simulink model "swingupcontroller"  (R2019b)
settings: Solver=VariableStepAuto  StartTime=0.0  StopTime=10.0  RelTol=1e-3
values from neighbouring files (symbols this model uses):
  epsilon = 12.0 * pi / 180    (= 0.209439510239)    [ripbalanced.m]    (also in setup_rotpen.m)
  eta_g = 0.90    (= 0.9)    [config_servo.m]    (also in dripbalanced.m; ripbalanced.m; test_drip.m)
  eta_m = 0.69    [config_servo.m]    (also in dripbalanced.m; ripbalanced.m; test_drip.m)
  g = 9.81    [RIP_ABCD_SS.m]    (also in RIP_ABCD_SS_1.m; RIP_ABCD_SS_2.m; RIP_ABCD_SS_3.m; RIP_ABCD_SS_POLE_PLACE.m)
  Jp = 0.001198    [RIP_ABCD_SS.m]    (also in RIP_ABCD_SS_2.m = 0.0023; RIP_ABCD_SS_3.m; RIP_ABCD_SS_POLE_PLACE.m; Untitled3.m = 0.0012)
  K = [0 0 0 0]    [Pole_placement.m]    (also in RIP_ABCD_SS.m = lqr(A,B,Q,R); RIP_ABCD_SS_POLE_PLACE.m = lqr(A,B,Q,R); ripbalanced.m = acker(A,B,DP); setup_rotpen.m = d_balance(A, B, zeta, wn, p3, p4))
  K_AMP = 1    [dripbalanced.m]    (also in ripbalanced.m; setup_rotpen.m; test_drip.m)
  Kg = 70    [RIP_ABCD_SS.m]    (also in RIP_ABCD_SS_1.m = 14; RIP_ABCD_SS_2.m; RIP_ABCD_SS_3.m; RIP_ABCD_SS_POLE_PLACE.m)
  km = 0.007677    [RIP_ABCD_SS.m]    (also in RIP_ABCD_SS_1.m = 0.00767; RIP_ABCD_SS_2.m = 0.00767; RIP_ABCD_SS_3.m; RIP_ABCD_SS_POLE_PLACE.m)
  kt = 0.007682    [RIP_ABCD_SS.m]    (also in RIP_ABCD_SS_1.m = 0.00767; RIP_ABCD_SS_2.m = 0.00767; RIP_ABCD_SS_3.m; RIP_ABCD_SS_POLE_PLACE.m)
  Lp = 0.33655    [RIP_ABCD_SS.m]    (also in RIP_ABCD_SS_1.m = 0.337; RIP_ABCD_SS_2.m = 0.6413; RIP_ABCD_SS_3.m; RIP_ABCD_SS_POLE_PLACE.m)
  Lr = 0.2159    [RIP_ABCD_SS.m]    (also in RIP_ABCD_SS_1.m = 0.216; RIP_ABCD_SS_2.m; RIP_ABCD_SS_3.m; RIP_ABCD_SS_POLE_PLACE.m)
  Mp = 0.127    [RIP_ABCD_SS.m]    (also in RIP_ABCD_SS_1.m; RIP_ABCD_SS_2.m = 0.23; RIP_ABCD_SS_3.m; RIP_ABCD_SS_POLE_PLACE.m)
  Mr = 0.257    [RIP_ABCD_SS.m]    (also in RIP_ABCD_SS_3.m; RIP_ABCD_SS_POLE_PLACE.m; dripbalanced.m; ripbalanced.m)
  Rm = 2.6    [RIP_ABCD_SS.m]    (also in RIP_ABCD_SS_1.m; RIP_ABCD_SS_2.m; RIP_ABCD_SS_3.m; RIP_ABCD_SS_POLE_PLACE.m)
libraries: simulink_extras x3, simulink x3
settings Model: Creator=Ridma  LastModifiedBy=Ridma

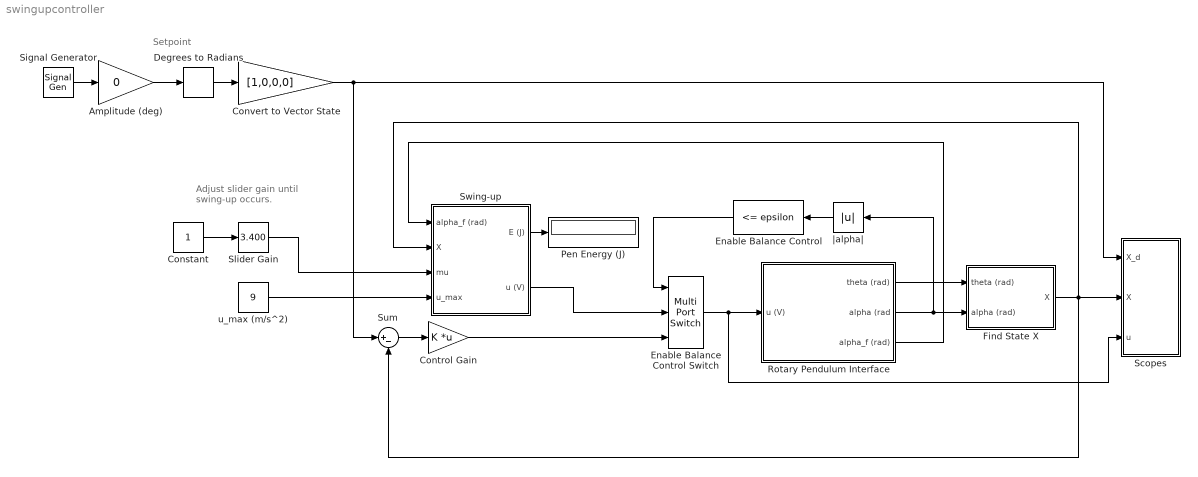
== system swingupcontroller ==
  note: Adjust slider gain
      | until swing-up occurs.
  note: Setpoint
  Amplitude (deg) : Gain  Gain=0  SaturateOnIntegerOverflow=on  OutDataTypeStr=Inherit: Same as input  ParamDataTypeStr=Inherit: Same as input
  Constant : Constant
  Control Gain : Gain  Gain=K  Multiplication=Matrix(K*u)
  Convert to Vector State : Gain  Gain=[1,0,0,0]
  Degrees to Radians : simulink_extras/Transformations/Degrees to Radians
  Enable Balance Control : simulink/Logic and Bit Operations/Compare To Constant  relop=<=  const=epsilon  OutDataTypeStr=uint8  ZeroCross=off
  Enable Balance Control Switch : MultiPortSwitch  DataPortOrder=Zero-based contiguous  Inputs=2  zeroidx=on
  Find State X : Subsystem
  Pen Energy (J) : Display
      settings: Decimation=100
  Rotary Pendulum Interface : Subsystem
  Scopes : Subsystem
  Signal Generator : SignalGenerator  WaveForm=square  Frequency=0.1
  Slider Gain : simulink/Math Operations/Slider Gain  gain=3.400  low=0  high=10
  Sum : Sum  Inputs=|+-
  Swing-up : Subsystem
  u_max (m/s^2) : Constant  Value=9
  |alpha| : Abs
  wires:
  Enable Balance Control Switch/1 -> Rotary Pendulum Interface/1(u (V)), Scopes/3(u)
  Control Gain/1 -> Enable Balance Control Switch/3
  Enable Balance Control/1 -> Enable Balance Control Switch/1
  Rotary Pendulum Interface/2(alpha (rad) -> Find State X/2(alpha (rad)), |alpha|/1
  Sum/1 -> Control Gain/1
  Constant/1 -> Slider Gain/1
  |alpha|/1 -> Enable Balance Control/1
  Rotary Pendulum Interface/3(alpha_f (rad)) -> Swing-up/1(alpha_f (rad))
  Swing-up/2(u (V)) -> Enable Balance Control Switch/2
  Slider Gain/1 -> Swing-up/3(mu)
  Swing-up/1(E (J)) -> Pen Energy (J)/1
  Signal Generator/1 -> Amplitude (deg)/1
  u_max (m/s^2)/1 -> Swing-up/4(u_max)
  Rotary Pendulum Interface/1(theta (rad)) -> Find State X/1(theta (rad))
  Find State X/1(X) -> Scopes/2(X), Sum/2, Swing-up/2(X)
  Convert to Vector State/1 -> Scopes/1(X_d), Sum/1
  Degrees to Radians/1 -> Convert to Vector State/1
  Amplitude (deg)/1 -> Degrees to Radians/1

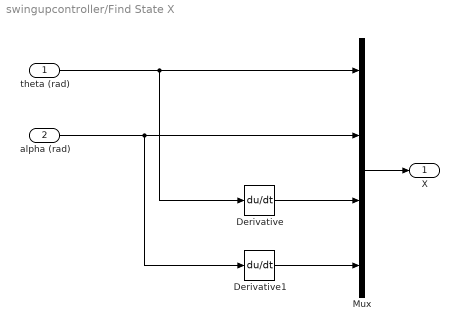
== system swingupcontroller/Find State X ==
  theta (rad) : Inport
  alpha (rad) : Inport  Port=2
  Derivative : Derivative
  Derivative1 : Derivative
  Mux : Mux
  X : Outport  VectorParamsAs1DForOutWhenUnconnected=off
  wires:
  alpha (rad)/1 -> Derivative1/1, Mux/2
  Mux/1 -> X/1
  theta (rad)/1 -> Derivative/1, Mux/1
  Derivative/1 -> Mux/3
  Derivative1/1 -> Mux/4

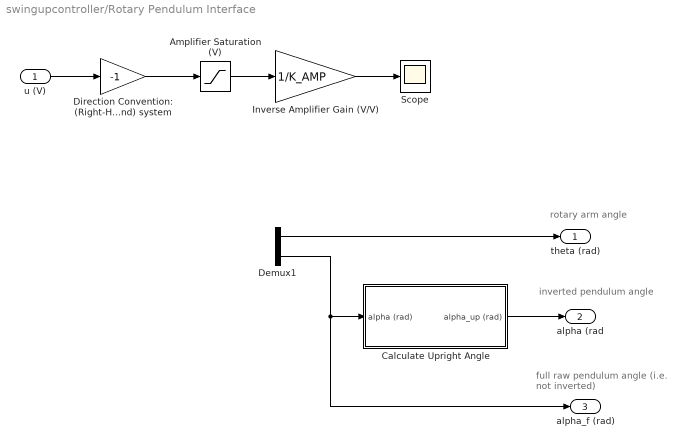
== system swingupcontroller/Rotary Pendulum Interface ==
  note: full raw pendulum angle
      |  (i.e. not inverted)
  note: rotary arm angle
  note: inverted pendulum angle
  u (V) : Inport
  Amplifier Saturation (V) : Saturate  UpperLimit=5  LowerLimit=-5
  Calculate Upright Angle : Subsystem
  Demux1 : Demux  Outputs=2
  Direction Convention: (Right-Hand) system : Gain  Gain=-1  SaturateOnIntegerOverflow=on  OutDataTypeStr=Inherit: Same as input  ParamDataTypeStr=Inherit: Same as input
  Inverse Amplifier Gain (V/V) : Gain  Gain=1/K_AMP
  Scope : Scope
  theta (rad) : Outport  VectorParamsAs1DForOutWhenUnconnected=off
  alpha (rad : Outport  Port=2  VectorParamsAs1DForOutWhenUnconnected=off
  alpha_f (rad) : Outport  Port=3  VectorParamsAs1DForOutWhenUnconnected=off
  wires:
  Calculate Upright Angle/1(alpha_up (rad)) -> alpha (rad/1
  Demux1/1 -> theta (rad)/1
  Direction Convention: (Right-Hand) system/1 -> Amplifier Saturation (V)/1
  u (V)/1 -> Direction Convention: (Right-Hand) system/1
  Inverse Amplifier Gain (V/V)/1 -> Scope/1
  Amplifier Saturation (V)/1 -> Inverse Amplifier Gain (V/V)/1
  Demux1/2 -> alpha_f (rad)/1, Calculate Upright Angle/1(alpha (rad))

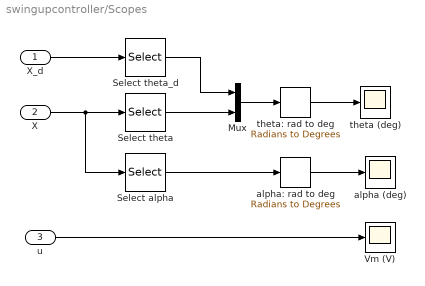
== system swingupcontroller/Scopes ==
  X_d : Inport
  X : Inport  Port=2
  u : Inport  Port=3
  Mux : Mux  Inputs=2
  Select alpha : Selector  InputPortWidth=4  IndexOptions=Index vector (dialog)  Indices=2  OutputSizes=[(-2)]
  Select theta : Selector  InputPortWidth=4  IndexOptions=Index vector (dialog)  Indices=1  OutputSizes=[(-2)]
  Select theta_d : Selector  InputPortWidth=4  IndexOptions=Index vector (dialog)  Indices=1  OutputSizes=[(-2)]
  Vm (V) : Scope
  alpha (deg) : Scope
  alpha: rad to deg : simulink_extras/Transformations/Radians to Degrees
  theta (deg) : Scope
  theta: rad to deg : simulink_extras/Transformations/Radians to Degrees
  wires:
  u/1 -> Vm (V)/1
  X_d/1 -> Select theta_d/1
  Mux/1 -> theta: rad to deg/1
  Select alpha/1 -> alpha: rad to deg/1
  alpha: rad to deg/1 -> alpha (deg)/1
  X/1 -> Select alpha/1, Select theta/1
  Select theta_d/1 -> Mux/1
  theta: rad to deg/1 -> theta (deg)/1
  Select theta/1 -> Mux/2

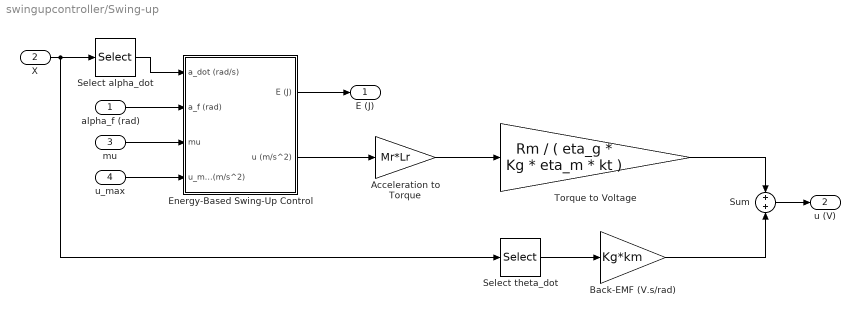
== system swingupcontroller/Swing-up ==
  alpha_f (rad) : Inport
  X : Inport  Port=2
  mu : Inport  Port=3
  u_max : Inport  Port=4
  Acceleration to Torque : Gain  Gain=Mr*Lr
  Back-EMF (V.s/rad) : Gain  Gain=Kg*km
  Energy-Based Swing-Up Control : Subsystem
  Select alpha_dot : Selector  InputPortWidth=4  IndexOptions=Index vector (dialog)  Indices=[4]  OutputSizes=1
  Select theta_dot : Selector  InputPortWidth=4  IndexOptions=Index vector (dialog)  Indices=[3]  OutputSizes=1
  Sum : Sum
  Torque to Voltage : Gain  Gain=Rm / ( eta_g * Kg * eta_m * kt )
  E (J) : Outport  VectorParamsAs1DForOutWhenUnconnected=off
  u (V) : Outport  Port=2  VectorParamsAs1DForOutWhenUnconnected=off
  wires:
  Energy-Based Swing-Up Control/2(u (m/s^2)) -> Acceleration to Torque/1
  Acceleration to Torque/1 -> Torque to Voltage/1
  Energy-Based Swing-Up Control/1(E (J)) -> E (J)/1
  alpha_f (rad)/1 -> Energy-Based Swing-Up Control/2(a_f (rad))
  mu/1 -> Energy-Based Swing-Up Control/3(mu)
  Select alpha_dot/1 -> Energy-Based Swing-Up Control/1(a_dot (rad/s))
  X/1 -> Select alpha_dot/1, Select theta_dot/1
  u_max/1 -> Energy-Based Swing-Up Control/4(u_max (m/s^2))
  Select theta_dot/1 -> Back-EMF (V.s/rad)/1
  Torque to Voltage/1 -> Sum/1
  Back-EMF (V.s/rad)/1 -> Sum/2
  Sum/1 -> u (V)/1

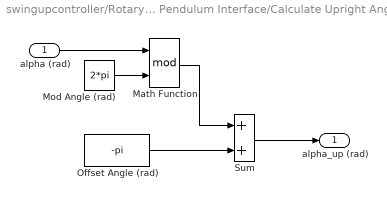
== system swingupcontroller/Rotary Pendulum Interface/Calculate Upright Angle ==
  alpha (rad) : Inport
  Math Function : Math  Operator=mod  SaturateOnIntegerOverflow=on
  Mod Angle (rad) : Constant  Value=2*pi
  Offset Angle (rad) : Constant  Value=-pi
  Sum : Sum  SaturateOnIntegerOverflow=on  InputSameDT=on  OutDataTypeStr=Inherit: Same as first input
  alpha_up (rad) : Outport  VectorParamsAs1DForOutWhenUnconnected=off
  wires:
  Math Function/1 -> Sum/1
  alpha (rad)/1 -> Math Function/1
  Offset Angle (rad)/1 -> Sum/2
  Mod Angle (rad)/1 -> Math Function/2
  Sum/1 -> alpha_up (rad)/1

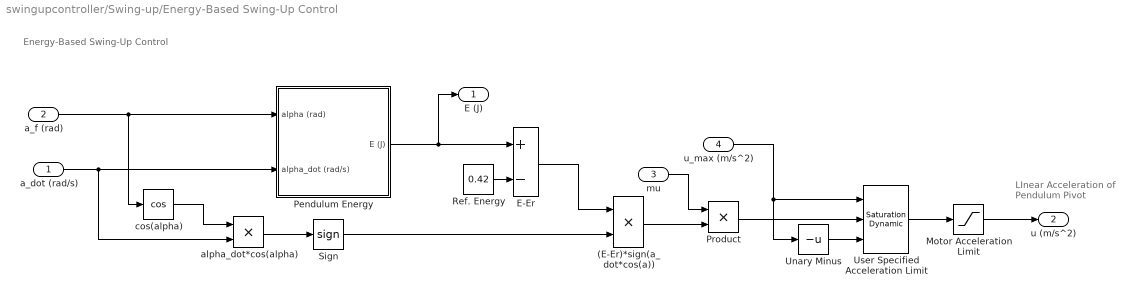
== system swingupcontroller/Swing-up/Energy-Based Swing-Up Control ==
  note: Energy-Based Swing-Up Control
  note: LInear Acceleration of
      | Pendulum Pivot
  a_dot (rad/s) : Inport
  a_f (rad) : Inport  Port=2
  mu : Inport  Port=3
  u_max (m/s^2) : Inport  Port=4
  (E-Er)*sign(a_dot*cos(a)) : Product  RndMeth=Zero
  E-Er : Sum  Inputs=+-
  Motor Acceleration Limit : Saturate  UpperLimit=9  LowerLimit=-9
  Pendulum Energy : Subsystem
  Product : Product  RndMeth=Zero
  Ref. Energy : Constant  Value=0.42
  Sign : Signum
  Unary Minus : UnaryMinus
  User Specified Acceleration Limit : simulink/Discontinuities/Saturation Dynamic  OutMin=[]  OutMax=[]  OutDataTypeStr=Inherit: Same as second input  OutDataType=fixdt(1, 16)  OutScaling=2^-10  DoSatur=off
  alpha_dot*cos(alpha) : Product  RndMeth=Zero
  cos(alpha) : Trigonometry  Operator=cos
  E (J) : Outport  VectorParamsAs1DForOutWhenUnconnected=off
  u (m/s^2) : Outport  Port=2  VectorParamsAs1DForOutWhenUnconnected=off
  wires:
  alpha_dot*cos(alpha)/1 -> Sign/1
  Sign/1 -> (E-Er)*sign(a_dot*cos(a))/2
  cos(alpha)/1 -> alpha_dot*cos(alpha)/1
  a_f (rad)/1 -> cos(alpha)/1, Pendulum Energy/1(alpha (rad))
  E-Er/1 -> (E-Er)*sign(a_dot*cos(a))/1
  Pendulum Energy/1(E (J)) -> E (J)/1, E-Er/1
  a_dot (rad/s)/1 -> alpha_dot*cos(alpha)/2, Pendulum Energy/2(alpha_dot (rad/s))
  (E-Er)*sign(a_dot*cos(a))/1 -> Product/2
  Ref. Energy/1 -> E-Er/2
  mu/1 -> Product/1
  Product/1 -> User Specified Acceleration Limit/2
  u_max (m/s^2)/1 -> User Specified Acceleration Limit/1, Unary Minus/1
  Unary Minus/1 -> User Specified Acceleration Limit/3
  User Specified Acceleration Limit/1 -> Motor Acceleration Limit/1
  Motor Acceleration Limit/1 -> u (m/s^2)/1

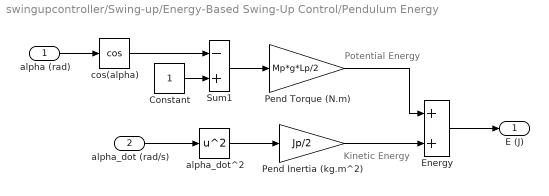
== system swingupcontroller/Swing-up/Energy-Based Swing-Up Control/Pendulum Energy ==
  note: Kinetic Energy
  note: Potential Energy
  alpha (rad) : Inport
  alpha_dot (rad/s) : Inport  Port=2
  Constant : Constant
  Energy : Sum  SaturateOnIntegerOverflow=on
  Pend Inertia (kg.m^2) : Gain  Gain=Jp/2
  Pend Torque (N.m) : Gain  Gain=Mp*g*Lp/2
  Sum1 : Sum  Inputs=-+  SaturateOnIntegerOverflow=on
  alpha_dot^2 : Math  Operator=square  SaturateOnIntegerOverflow=on
  cos(alpha) : Trigonometry  Operator=cos
  E (J) : Outport  VectorParamsAs1DForOutWhenUnconnected=off
  wires:
  Constant/1 -> Sum1/2
  Pend Inertia (kg.m^2)/1 -> Energy/2
  Sum1/1 -> Pend Torque (N.m)/1
  alpha_dot^2/1 -> Pend Inertia (kg.m^2)/1
  Pend Torque (N.m)/1 -> Energy/1
  alpha (rad)/1 -> cos(alpha)/1
  alpha_dot (rad/s)/1 -> alpha_dot^2/1
  Energy/1 -> E (J)/1
  cos(alpha)/1 -> Sum1/1
